simulink model "motore_osservatore_s"  (R2018b)
settings: Solver=VariableStepAuto  StartTime=0.0  StopTime=10.0  RelTol=1e-3
values from neighbouring files (symbols this model uses):
  A = [-11 -2.5 0;4 0 0;0 0.25 0]    [ex1.m]    (also in ex2.m; ex3.m = sys_s.a; ex4.m = sys_s.A; ex5.m = sys_c.A)
  B = [4 0 0]'    [ex1.m]    (also in ex2.m; ex3.m = sys_s.b; ex4.m = sys_s.B; ex5.m = sys_c.B)
  C = [0 0 5]    [ex1.m]    (also in ex2.m; ex3.m = sys_s.c; ex4.m = sys_s.C; ex5.m = sys_c.C)
  H = -acker(A',C',[lam_o lam_o lam_o*10])'    [ex7.m]    (also in ex8.m; motore.m = -acker(A',C',[lam_o lam_o])'; motore_posizione.m = -acker(A',C',[lam_o1 lam_o2 lam_o1])')
  K = -acker(A,B,lam_d)    [ex1.m]    (also in ex2.m; ex3.m = -acker(A,B,lam_ds); ex4.m; ex5.m)
  k_w = k_d/k_F    [ex2.m]    (also in ex3.m; ex4.m; ex5.m; ex6.m)
settings Model: Creator=michelemaresca  LastModifiedBy=michelemaresca

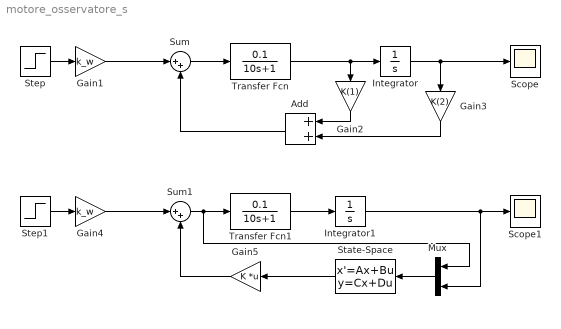
== system motore_osservatore_s ==
  Add : Sum
  Gain1 : Gain  Gain=k_w
  Gain2 : Gain  Gain=K(1)
  Gain3 : Gain  Gain=K(2)
  Gain4 : Gain  Gain=k_w
  Gain5 : Gain  Gain=K  Multiplication=Matrix(K*u)
  Integrator : Integrator
  Integrator1 : Integrator
  Mux : Mux  Inputs=2
  Scope : Scope
  Scope1 : Scope
  State-Space : StateSpace  A=A+H*C  B=[B -H]  C=eye(2)  D=zeros(2,2)  InitialCondition=0
  Step : Step  Time=0  SampleTime=0
  Step1 : Step  Time=0  SampleTime=0
  Sum : Sum  Inputs=|++
  Sum1 : Sum  Inputs=|++
  Transfer Fcn : TransferFcn  Numerator=[0.1]  Denominator=[10 1]
  Transfer Fcn1 : TransferFcn  Numerator=[0.1]  Denominator=[10 1]
  wires:
  Step/1 -> Gain1/1
  Gain1/1 -> Sum/1
  Sum/1 -> Transfer Fcn/1
  Add/1 -> Sum/2
  Transfer Fcn/1 -> Gain2/1, Integrator/1
  Integrator/1 -> Gain3/1, Scope/1
  Gain2/1 -> Add/1
  Gain3/1 -> Add/2
  Step1/1 -> Gain4/1
  State-Space/1 -> Gain5/1
  Transfer Fcn1/1 -> Integrator1/1
  Gain4/1 -> Sum1/1
  Integrator1/1 -> Mux/2, Scope1/1
  Sum1/1 -> Mux/1, Transfer Fcn1/1
  Gain5/1 -> Sum1/2
  Mux/1 -> State-Space/1
